simulink model "pendule_inv_etu"  (R2019a)
settings: Solver=VariableStepAuto  StartTime=0.0  StopTime=10.0  RelTol=1e-3
values from neighbouring files (symbols this model uses):
  g = 9.81    [simu_pendule_inv_capteur_etu.m]    (also in simu_pendule_inv_echant_etu.m; simu_pendule_inv_etu.m)
  K = [10 1]    [simu_pendule_inv_capteur_etu.m]    (also in simu_pendule_inv_echant_etu.m = [30 10]; simu_pendule_inv_etu.m = [30 10])
  l = 10    [simu_pendule_inv_capteur_etu.m]    (also in simu_pendule_inv_echant_etu.m; simu_pendule_inv_etu.m)
  ue = 0    [simu_pendule_inv_capteur_etu.m]    (also in simu_pendule_inv_echant_etu.m; simu_pendule_inv_etu.m)
  x0 = [pi/20 0]'    [simu_pendule_inv_capteur_etu.m]    (also in simu_pendule_inv_echant_etu.m; simu_pendule_inv_etu.m = [pi/10 0]')
  xe = [0 0]'    [simu_pendule_inv_capteur_etu.m]    (also in simu_pendule_inv_echant_etu.m; simu_pendule_inv_etu.m)
settings Model: Creator=aakby  LastModifiedBy=hmoudden

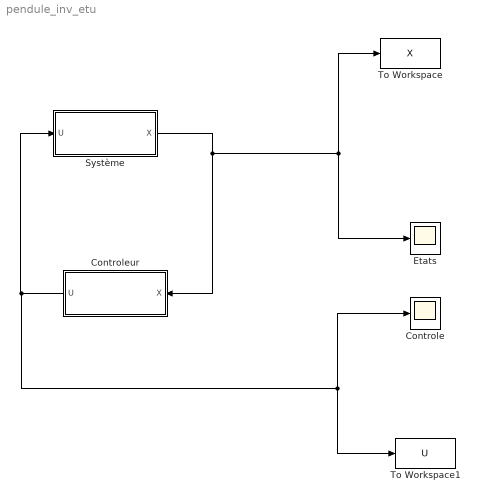
== system pendule_inv_etu ==
  Controle : Scope
  Controleur : Subsystem
  Etats : Scope
  Système : Subsystem
  To Workspace : ToWorkspace  VariableName=X  SaveFormat=Timeseries  SampleTime=-1
  To Workspace1 : ToWorkspace  VariableName=U  SaveFormat=Timeseries  SampleTime=-1
  wires:
  Système/1(X) -> Controleur/1(X), Etats/1, To Workspace/1
  Controleur/1(U) -> To Workspace1/1, Controle/1, Système/1(U)

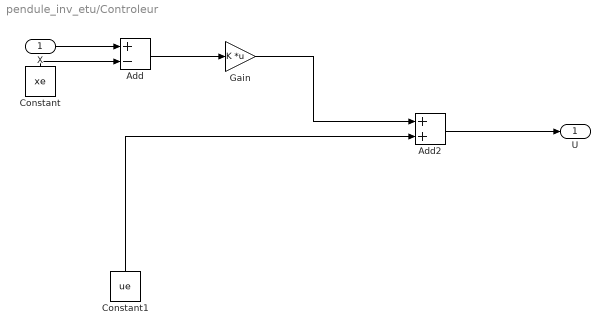
== system pendule_inv_etu/Controleur ==
  X : Inport
  Add : Sum  Inputs=+-
  Add2 : Sum
  Constant : Constant  Value=xe
  Constant1 : Constant  Value=ue
  Gain : Gain  Gain=K  Multiplication=Matrix(K*u)
  U : Outport
  wires:
  X/1 -> Add/1
  Constant/1 -> Add/2
  Add/1 -> Gain/1
  Gain/1 -> Add2/1
  Constant1/1 -> Add2/2
  Add2/1 -> U/1

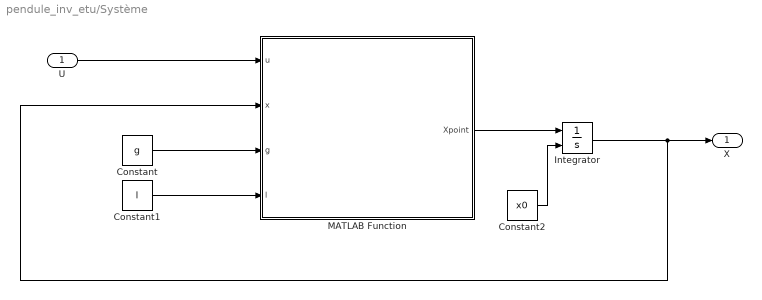
== system pendule_inv_etu/Système ==
  U : Inport
  Constant : Constant  Value=g
  Constant1 : Constant  Value=l
  Constant2 : Constant  Value=x0
  Integrator : Integrator  InitialConditionSource=external
  MATLAB Function : MATLAB Function  TreatAsAtomicUnit=on
  X : Outport
  wires:
  U/1 -> MATLAB Function/1(u)
  MATLAB Function/1(Xpoint) -> Integrator/1
  Integrator/1 -> X/1, MATLAB Function/2(x)
  Constant1/1 -> MATLAB Function/4(l)
  Constant/1 -> MATLAB Function/3(g)
  Constant2/1 -> Integrator/2

== matlab function pendule_inv_etu/Système/MATLAB Function ==
  data: u input; Xpoint output; x input; g input; l input
function Xpoint = fcn(u,x,g,l)

Xpoint = [x(2) g/l*sin(x(1))-cos(x(1))*u/l]';
